simulink model "NA3_proportional_saturation_regul"  (R2024b)
settings: Solver=VariableStepAuto  StartTime=0.0  StopTime=T_SIM  MaxStep=0.001  RelTol=1e-3
values from neighbouring files (symbols this model uses):
  control_par = [k_1, k_2, k_3]    [init_regulation.m]
  controller_index = 2    [init_regulation.m]
  d = d_nominal    (= 0.165)    [init_regulation.m]
  d_actual = d_nominal    (= 0.165)    [init_regulation.m]
  omega_M = 12    [init_regulation.m]
  q_d = [2;2;0]    [init_regulation.m]
  Q_INIT = [0;0;0]    [init_regulation.m]
  r = r_nominal    (= 0.03)    [init_regulation.m]
  r_actual = r_nominal    (= 0.03)    [init_regulation.m]
settings Model: Creator=alber  LastModifiedBy=Enrico
settings RTWCC: GPUComputeCapability=3.5

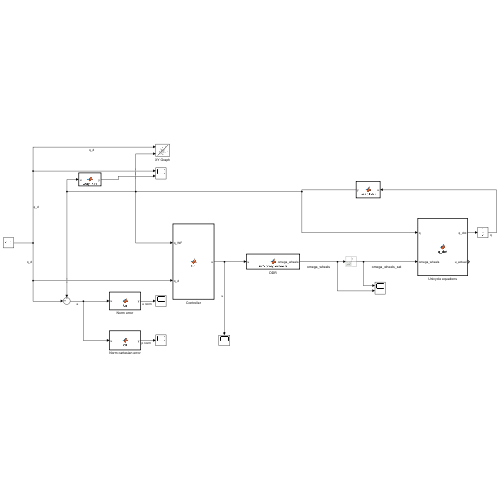
[thumbnail: Simulink's stored preview of the top-level diagram]
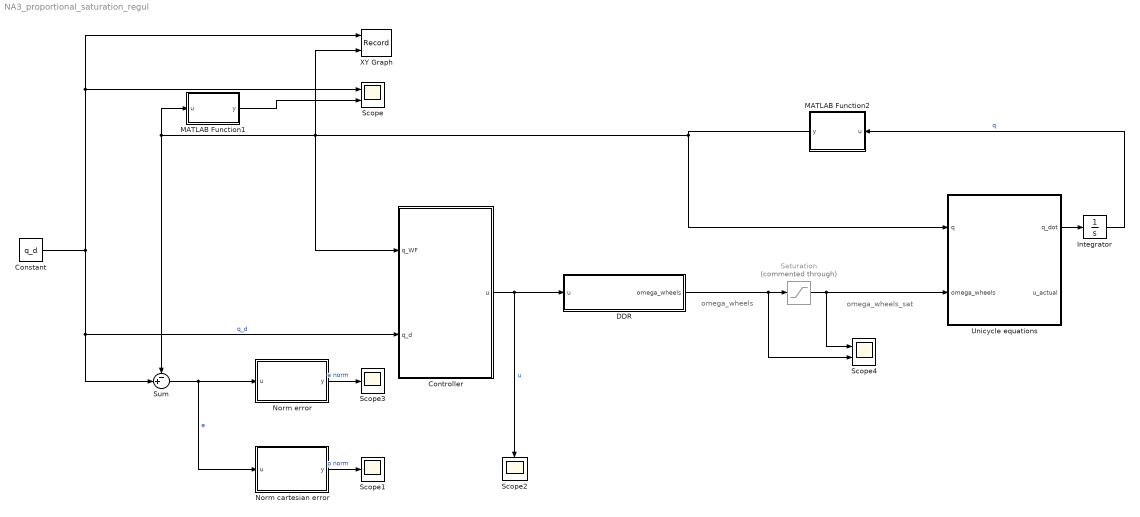
== system NA3_proportional_saturation_regul ==
  note: omega_wheels_sat
  note: omega_wheels
  Constant : Constant  Value=q_d
  Controller : MATLAB Function  TreatAsAtomicUnit=on
  DDR : MATLAB Function  TreatAsAtomicUnit=on
  Integrator : Integrator  InitialCondition=Q_INIT
  MATLAB Function1 : MATLAB Function  TreatAsAtomicUnit=on
  MATLAB Function2 : MATLAB Function  TreatAsAtomicUnit=on
  Norm cartesian error : MATLAB Function  TreatAsAtomicUnit=on
  Norm error : MATLAB Function  TreatAsAtomicUnit=on
  Saturation : Saturate  Commented=through  UpperLimit=omega_M  LowerLimit=-omega_M
  Scope : Scope  NumInputPorts=2
  Scope1 : Scope
  Scope2 : Scope
  Scope3 : Scope
  Scope4 : Scope  NumInputPorts=2
  Sum : Sum  Inputs=-+|
  Unicycle equations : MATLAB Function  TreatAsAtomicUnit=on
  XY Graph : Record  FileSettingsInternal="{\"entries\":[{\"content\":{\"excelSettings\":{\"content\":{},\"type\":\"Streamout.ExcelSettings\"}},\"type\":\"Streamout.FileSettingStorage\",\"uuid\":\"\"}],\"packageUris\":[\"http:\\/\\/schema.mathworks.com\\/mf0\\/streamout_blocks\\/R2020a\"],\"version\":\"1.0\"}"  Layout=[1 2]  SignalsInternal="{\"entries\":[{\"content\":{\"signals\":[{\"content\":{\"blockPath\":[],\"dimensions\":[3,1],\"domain\":\"\",\"hasChildren\":true,\"lineColor\":\"#edb120\",\"lineWidth\":2,\"port\":2,\"sid\":[\"\"],\"signalID\":1,\"signalName\":\"MATLAB Function2\"},\"type\":\"RecordBlkView.Signal\",\"uuid\":\"\"},{\"content\":{\"blockPath\":[],\"channel\":[1,1],\"dimensions\":[3,1],\"domain\":\"\",\"lineColor\":\"#000000\",\"lineStyle\":\"DASH_DOT\",\"parentID\":1,\"plots\":[ 1 ],\"port\":2,\"sid\":[\"\"],\"signalID\":2,\"signalName\":\"MATLAB Function2\"},\"type\":\"RecordBlkView.Signal\",\"uuid\":\"\"},{\"content\":{\"blockPath\":[],\"dimensions\":[3],\"domain\":\"\",\"hasChildren\":true,\"lineColor\":\"#77ac30\",\"lineWidth\":2,\"port\":1,\"sid\":[\"\"],\"signalID\":3,\"signalName\":\"q_d\"},\"type\":\"RecordBlkView.Signal\",\"uuid\":\"\"},{\"content\":{\"blockPath\":[],\"channel\":[1],\"dimensions\":[3],\"domain\":\"\",\"lineColor\":\"#d95319\",\"parentID\":3,\"plots\":[ 1 ],\"port\":1,\"sid\":[\"\"],\"signalID\":4,\"signalName\":\"q_d\"},\"type\":\"RecordBlkView.Signal\",\"uuid\":\"\"},{\"content\":{\"blockPath\":[],\"channel\":[2,1],\"dimensions\":[3,1],\"domain\":\"\",\"lineColor\":\"#edb120\",\"lineWidth\":2,\"parentID\":1,\"plots\":[ 1 ],\"port\":2,\"sid\":[\"\"],\"signalID\":5,\"signalName\":\"MATLAB Function2\"},\"type\":\"RecordBlkView.Signal\",\"uuid\":\"\"},{\"content\":{\"blockPath\":[],\"channel\":[3,1],\"dimensions\":[3,1],\"domain\":\"\",\"lineColor\":\"#7e2f8e\",\"lineWidth\":2,\"parentID\":1,\"plots\":[ 2, 9 ],\"port\":2,\"sid\":[\"\"],\"signalID\":6,\"signalName\":\"MATLAB Function2\"},\"type\":\"RecordBlkView.Signal\",\"uuid\":\"\"},{\"content\":{\"blockPath\":[],\"channel\":[2],\"dimensions\":[3],\"domain\":\"\",\"lineColor\":\"#77ac30\",\"parentID\":3,\"plots\":[ 1 ],\"port\":1,\"sid\":[\"\"],\"signalID\":7,\"signalName\":\"q_d\"},\"type\":\"RecordBlkView.Signal\",\"uuid\":\"\"},{\"content\":{\"blockPath\":[],\"channel\":[3],\"dimensions\":[3],\"domain\":\"\",\"lineColor\":\"#4dbeee\",\"parentID\":3,\"plots\":[ 2, 9 ],\"port\":1,\"sid\":[\"\"],\"signalID\":8,\"signalName\":\"q_d\"},\"type\":\"RecordBlkView.Signal\",\"uuid\":\"\"}]},\"type\":\"RecordBlkView.InputSignals\",\"uuid\":\"\"}],\"packageUris\":[\"http:\\/\\/schema.mathworks.com\\/mf0\\/streamout_blocks\\/R2020a\"],\"version\":\"1.0\"}"  VisualizationBindings="{\"xyplotplugin\":{\"info\":[{\"series\":[{\"bindingParametersList\":[{\"parameter\":\"X-Axis\",\"signalID\":4,\"signalName\":\"q_d(1)\"},{\"parameter\":\"Y-Axis\",\"signalID\":7,\"signalName\":\"q_d(2)\"}],\"seriesID\":0},{\"bindingParametersList\":[{\"parameter\":\"X-Axis\",\"signalID\":2,\"signalName\":\"MATLAB Function2(1,1)\"},{\"parameter\":\"Y-Axis\",\"signalID\":5,\"signalName\":\"MATLAB Function2(2,1)\"}],\"seriesID\":1}],\"subplotID\":1}]}}"  CompatibilityTag=XY
  wires:
  Integrator/1 -> MATLAB Function2/1(u)  "q"
  Unicycle equations/1(q_dot) -> Integrator/1
  Constant/1 -> Sum/2, Controller/2(q_d), XY Graph/1, Scope/1  "q_d"
  Sum/1 -> Norm cartesian error/1(u), Norm error/1(u)  "e"
  Controller/1(u) -> DDR/1(u), Scope2/1  "u"
  Norm cartesian error/1(y) -> Scope1/1  "p norm"
  DDR/1(omega_wheels) -> Saturation/1, Scope4/2
  Saturation/1 -> Unicycle equations/2(omega_wheels), Scope4/1
  Norm error/1(y) -> Scope3/1  "e norm"
  MATLAB Function2/1(y) -> Sum/1, MATLAB Function1/1(u), Controller/1(q_WF), XY Graph/2, Unicycle equations/1(q)
  MATLAB Function1/1(y) -> Scope/2

== matlab function NA3_proportional_saturation_regul/Norm cartesian error ==
  data: u input; y output
function y = fcn(u)

y = sqrt(sum(u(1:2).^2));

== matlab function NA3_proportional_saturation_regul/Unicycle equations ==
  data: q input; omega_wheels input; q_dot output; r_actual parameter; d_actual parameter; u_actual output
function [q_dot, u_actual] = q_dot(q, omega_wheels, r_actual, d_actual)
u_actual = [r_actual/2, r_actual/2;-r_actual/d_actual, r_actual/d_actual]*omega_wheels;
theta = q(3);
q_dot = [[cos(theta), 0];[sin(theta), 0];[0,1]]*u_actual;

== matlab function NA3_proportional_saturation_regul/Norm error ==
  data: u input; y output
function y = fcn(u)
y = [u(1);u(2); wrapToPi(u(3))];

== matlab function NA3_proportional_saturation_regul/Controller ==
  data: q_WF input; q_d input; u output; controller_index parameter; control_par parameter
function u = fcn(q_WF, q_d, controller_index, control_par)

% roto translation
omega_d = q_d(3);
e = q_WF - q_d;
q_WF(1) = cos(omega_d)*e(1) + sin(omega_d)*e(2);
q_WF(2) = -sin(omega_d)*e(1) + cos(omega_d)*e(2);
q_WF(3) = e(3);


% select the controller
if controller_index == 1
    % cartesian regulator
    % transform q_WF
    % compute the input
    e_p = [-q_WF(1); -q_WF(2)];
    n = [cos(q_WF(3)); sin(q_WF(3))];
    % pointing error
    gamma = wrapToPi(atan2(q_WF(2),q_WF(1)) + pi - q_WF(3));

    v = control_par(1) * (e_p' * n);
    omega = control_par(2) * gamma;
    u = [v;omega];

else
    % posture regulator
    % transform q_WF
    % compute pointing error

    ro = sqrt(q_WF(1)^2 + q_WF(2)^2);
    % pointing error
    gamma = wrapToPi(atan2(q_WF(2),q_WF(1)) + pi - q_WF(3));
    delta = wrapToPi(gamma + q_WF(3));
    
    v = control_par(1) * ro * cos(gamma);

    if abs(gamma)<1e-4
        omega = control_par(2)*gamma + control_par(1)*cos(gamma)*(gamma + control_par(3)*delta);
    else
        omega = control_par(2)*gamma + control_par(1)*sin(gamma)*cos(gamma)*(gamma + control_par(3)*delta)/gamma;
    end
    
    u = [v;omega];
end

== matlab function NA3_proportional_saturation_regul/DDR ==
  data: u input; omega_wheels output; r parameter; d parameter; omega_M parameter
function omega_wheels = kin2omegawheels(u, r, d, omega_M)
omega_l = u(1)/r-d/(2*r)*u(2);
omega_r = u(1)/r+d/(2*r)*u(2);

if (abs(omega_l) > omega_M) || (abs(omega_r) > omega_M)
    omega_prop = max(abs(omega_l), abs(omega_r));
    omega_l = omega_l*omega_M/omega_prop;
    omega_r = omega_r*omega_M/omega_prop;
end
omega_wheels = [omega_l;omega_r];

== matlab function NA3_proportional_saturation_regul/MATLAB Function2 ==
  data: u input; y output
function y  = wrapToPi(u)
%theta = wrapToPi(u(3));
%theta = unwrap(u(3));
theta = u(3);
y = [u(1),u(2),theta]';

== matlab function NA3_proportional_saturation_regul/MATLAB Function1 ==
  data: u input; y output
function y  = wrapToPi(u)
%theta = wrapToPi(u(3));
%theta = unwrap(u(3));
theta = u(3);
y = [u(1),u(2),theta]';
